simulink model "Question1Sim"  (R2021b)
settings: Solver=VariableStepAuto  StartTime=0.0  StopTime=70  RelTol=1e-3
settings Model: Creator=Ali  LastModifiedBy=Matin

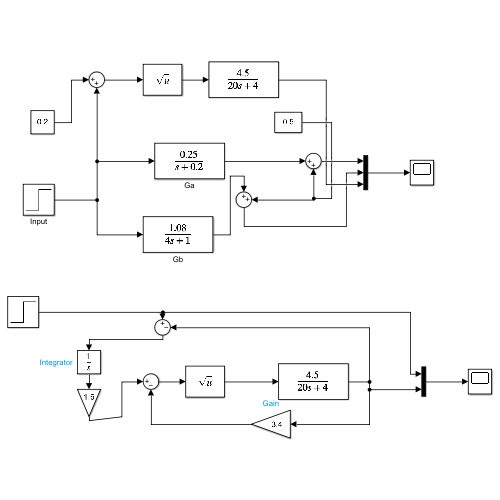
[thumbnail: Simulink's stored preview of the top-level diagram]
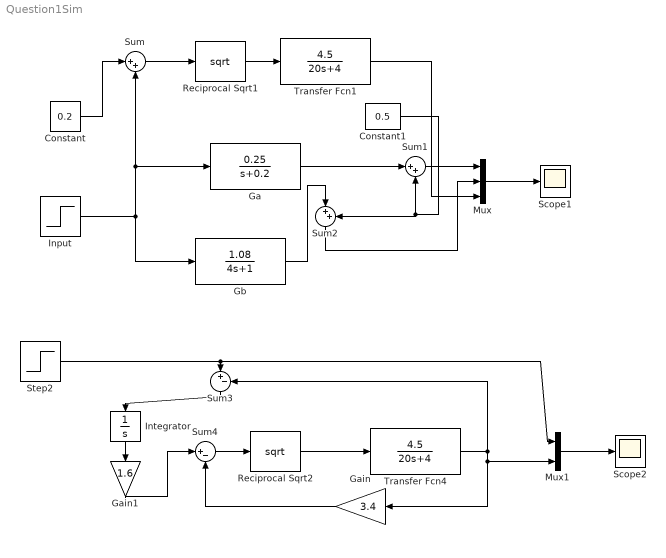
== system Question1Sim ==
  Constant : Constant  Value=0.2
  Constant1 : Constant  Value=0.5
  Ga : TransferFcn  Numerator=[0.25]  Denominator=[1 0.2]
  Gain : Gain  Gain=3.4
  Gain1 : Gain  Gain=1.6
  Gb : TransferFcn  Numerator=[1.08]  Denominator=[4 1]
  Input : Step  Time=30  After=0.05  SampleTime=0
  Integrator : Integrator
  Mux : Mux  Inputs=3
  Mux1 : Mux  Inputs=2
  Reciprocal Sqrt1 : Sqrt  SaturateOnIntegerOverflow=on
  Reciprocal Sqrt2 : Sqrt  SaturateOnIntegerOverflow=on
  Scope1 : Scope
  Scope2 : Scope
  Step2 : Step  Time=30  Before=0.5  After=0.6  SampleTime=0
  Sum : Sum  Inputs=|++
  Sum1 : Sum  Inputs=|++
  Sum2 : Sum  Inputs=|++
  Sum3 : Sum  Inputs=|+-
  Sum4 : Sum  Inputs=|+-
  Transfer Fcn1 : TransferFcn  Numerator=[4.5]  Denominator=[20 4]
  Transfer Fcn4 : TransferFcn  Numerator=[4.5]  Denominator=[20 4]
  wires:
  Reciprocal Sqrt1/1 -> Transfer Fcn1/1
  Sum/1 -> Reciprocal Sqrt1/1
  Constant/1 -> Sum/1
  Input/1 -> Ga/1, Sum/2, Gb/1
  Mux/1 -> Scope1/1
  Ga/1 -> Sum1/1
  Sum1/1 -> Mux/1
  Constant1/1 -> Sum2/2, Sum1/2
  Gb/1 -> Sum2/1
  Sum2/1 -> Mux/2
  Transfer Fcn4/1 -> Mux1/2, Gain/1, Sum3/2
  Sum4/1 -> Reciprocal Sqrt2/1
  Reciprocal Sqrt2/1 -> Transfer Fcn4/1
  Step2/1 -> Mux1/1, Sum3/1
  Sum3/1 -> Integrator/1
  Integrator/1 -> Gain1/1
  Gain1/1 -> Sum4/1
  Gain/1 -> Sum4/2
  Mux1/1 -> Scope2/1
  Transfer Fcn1/1 -> Mux/3
